simulink library "csc_gal_gdn_approach_landing_mtv_lib"  (R2014b)
settings: Solver=ode45  StartTime=0.0  StopTime=10.0  RelTol=1e-3
libraries: util_quat_lib x4, util_info_lib x1, util_common_lib x1, csc_lac_landing_acceleration_command_mtv_lib x1, csu_arg_aimpoint_roll_guidance_lib x1
settings Model: Creator=Nilesh  LastModifiedBy=tgorton

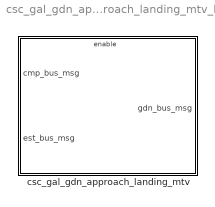
== system csc_gal_gdn_approach_landing_mtv_lib ==
  csc_gal_gdn_approach_landing_mtv : Subsystem

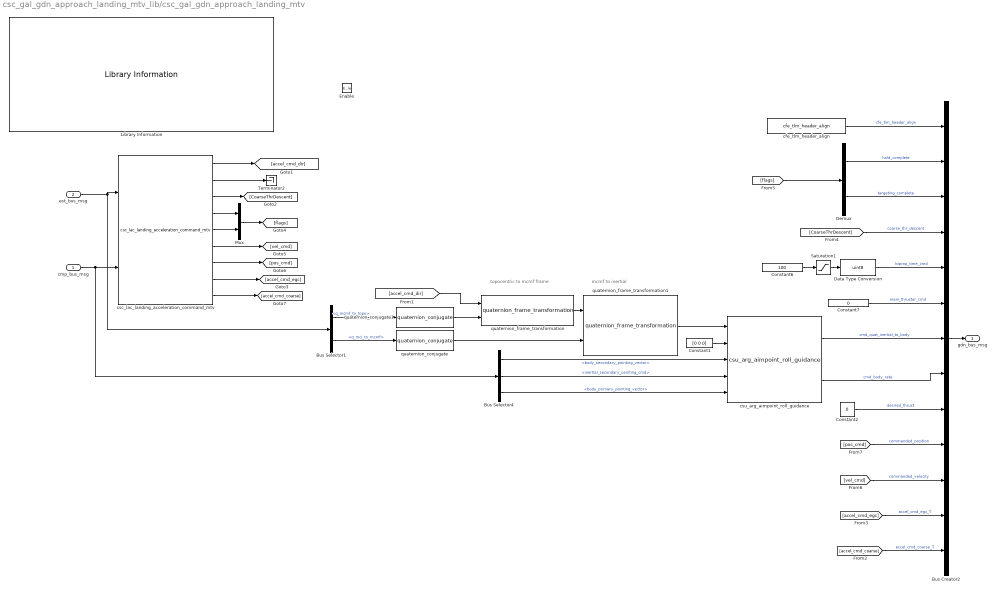
== system csc_gal_gdn_approach_landing_mtv_lib/csc_gal_gdn_approach_landing_mtv ==
  note: mcmf to inertial
  note: topocentric to mcmf frame
  cmp_bus_msg : Inport
  est_bus_msg : Inport  Port=2
  Enable : EnablePort
  Bus Selector1 : BusSelector  OutputSignals=q_mcmf_to_topo,q_mci_to_mcmf
  Bus Selector4 : BusSelector  OutputSignals=body_secondary_pointing_vector,inertial_secondary_pointing_cmd,body_primary_pointing_vector
  Bus Creator2 : BusCreator  Inputs=13  OutDataTypeStr=Bus: gdn_bus_msg  NonVirtualBus=on
  Constant1 : Constant  Value=[0 0 0]  SampleTime=-1
  Constant2 : Constant  Value=0
  Constant6 : Constant  Value=100
  Constant7 : Constant  Value=0
  Data Type Conversion : DataTypeConversion  OutDataTypeStr=uint8
  Demux : Demux  Outputs=2
  Library Information : util_info_lib/Library Information  owner='NONE'
  Mux : Mux  Inputs=2
  Saturation1 : Saturate  UpperLimit=100  LowerLimit=0
  Terminator2 : Terminator
  cfe_tlm_header_align : util_common_lib/cfe_tlm_header_align
  csc_lac_landing_acceleration_command_mtv : csc_lac_landing_acceleration_command_mtv_lib/csc_lac_landing_acceleration_command_mtv
  csu_arg_aimpoint_roll_guidance : csu_arg_aimpoint_roll_guidance_lib/csu_arg_aimpoint_roll_guidance
  quaternion_conjugate : util_quat_lib/quaternion_conjugate  SystemSampleTime=-1
  quaternion_conjugate1 : util_quat_lib/quaternion_conjugate  SystemSampleTime=-1
  quaternion_frame_transformation : util_quat_lib/quaternion_frame_transformation  SystemSampleTime=-1
  quaternion_frame_transformation1 : util_quat_lib/quaternion_frame_transformation  SystemSampleTime=-1
  gdn_bus_msg : Outport  OutDataTypeStr=Bus: gdn_bus_msg
  wires:
  [accel_cmd_coarse] -> Bus Creator2/13  "accel_cmd_coarse_T"
  [accel_cmd_egc] -> Bus Creator2/12  "accel_cmd_egc_T"
  csc_lac_landing_acceleration_command_mtv/8 -> [accel_cmd_egc]
  csc_lac_landing_acceleration_command_mtv/9 -> [accel_cmd_coarse]
  [accel_cmd_dir] -> quaternion_frame_transformation/1
  csc_lac_landing_acceleration_command_mtv/1 -> [accel_cmd_dir]
  csc_lac_landing_acceleration_command_mtv/2 -> Terminator2/1
  Constant6/1 -> Saturation1/1
  [pos_cmd] -> Bus Creator2/10  "commanded_position"
  [vel_cmd] -> Bus Creator2/11  "commanded_velocity"
  csc_lac_landing_acceleration_command_mtv/7 -> [pos_cmd]
  csc_lac_landing_acceleration_command_mtv/6 -> [vel_cmd]
  Data Type Conversion/1 -> Bus Creator2/5  "biprop_time_cmd"
  cfe_tlm_header_align/1 -> Bus Creator2/1  "cfe_tlm_header_align"
  csc_lac_landing_acceleration_command_mtv/5 -> Mux/2
  csc_lac_landing_acceleration_command_mtv/4 -> Mux/1
  Demux/1 -> Bus Creator2/2  "hold_complete"
  Demux/2 -> Bus Creator2/3  "targeting_complete"
  [flags] -> Demux/1
  Mux/1 -> [flags]
  Bus Selector1/2 -> quaternion_conjugate/1  "<q_mci_to_mcmf>"
  Bus Selector1/1 -> quaternion_conjugate1/1  "<q_mcmf_to_topo>"
  Bus Selector4/1 -> csu_arg_aimpoint_roll_guidance/3  "<body_secondary_pointing_vector>"
  csu_arg_aimpoint_roll_guidance/2 -> Bus Creator2/8  "cmd_body_rate"
  csu_arg_aimpoint_roll_guidance/1 -> Bus Creator2/7  "cmd_quat_inertial_to_body"
  quaternion_frame_transformation1/1 -> csu_arg_aimpoint_roll_guidance/1
  Bus Creator2/1 -> gdn_bus_msg/1
  quaternion_conjugate/1 -> quaternion_frame_transformation1/2
  quaternion_conjugate1/1 -> quaternion_frame_transformation/2
  Constant7/1 -> Bus Creator2/6  "main_thruster_cmd"
  quaternion_frame_transformation/1 -> quaternion_frame_transformation1/1
  cmp_bus_msg/1 -> csc_lac_landing_acceleration_command_mtv/2, Bus Selector4/1
  est_bus_msg/1 -> csc_lac_landing_acceleration_command_mtv/1, Bus Selector1/1
  Constant1/1 -> csu_arg_aimpoint_roll_guidance/2
  Bus Selector4/3 -> csu_arg_aimpoint_roll_guidance/5  "<body_primary_pointing_vector>"
  csc_lac_landing_acceleration_command_mtv/3 -> [CoarseThrDescent]
  [CoarseThrDescent] -> Bus Creator2/4  "coarse_thr_descent"
  Constant2/1 -> Bus Creator2/9  "desired_thrust"
  Bus Selector4/2 -> csu_arg_aimpoint_roll_guidance/4  "<inertial_secondary_pointing_cmd>"
  Saturation1/1 -> Data Type Conversion/1
